simulink model "robot_echant_etu"  (R2022a)
settings: Solver=VariableStepAuto  StartTime=0.0  StopTime=10.0  RelTol=1e-3
values from neighbouring files (symbols this model uses):
  K = -place(A,B,[-136.4009, -2.6408, -3.5890, -5.9800])    [matrices.m]    (also in simu_robot_etu.m = [0.6700 19.9055 1.0747  1.9614])
  ue = 0    [simu_robot_etu.m]
  x0 = [0 pi/10 0 0]    [simu_robot_etu.m]
  xe = [0 0 0 0]'    [simu_robot_etu.m]
undefined symbols (not defined in the file or in its folder): DiscIntNeverNeededParam, X0
libraries: simulink x1
settings Model: Creator=melallem  LastModifiedBy=elgue
settings DebuggingCC: UnconnectedInputMsg=warning  UnconnectedOutputMsg=warning  UnconnectedLineMsg=warning
settings RTWCC: DLArmComputeVersion=19.05

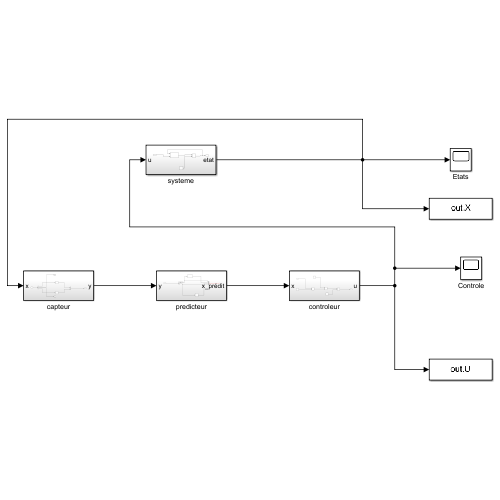
[thumbnail: Simulink's stored preview of the top-level diagram]
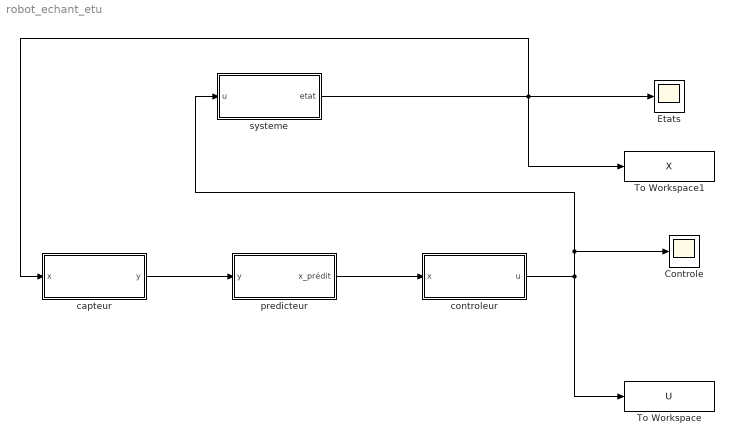
== system robot_echant_etu ==
  Controle : Scope
  Etats : Scope
  To Workspace : ToWorkspace  VariableName=U  SaveFormat=Timeseries  SampleTime=-1
  To Workspace1 : ToWorkspace  VariableName=X  SaveFormat=Timeseries  SampleTime=-1
  capteur : Subsystem
  controleur : Subsystem
  predicteur : Subsystem
  systeme : Subsystem
  wires:
  controleur/1(u) -> To Workspace/1, systeme/1(u), Controle/1
  predicteur/1(x_prédit) -> controleur/1(x)
  capteur/1(y) -> predicteur/1(y)
  systeme/1(etat) -> To Workspace1/1, capteur/1(x), Etats/1

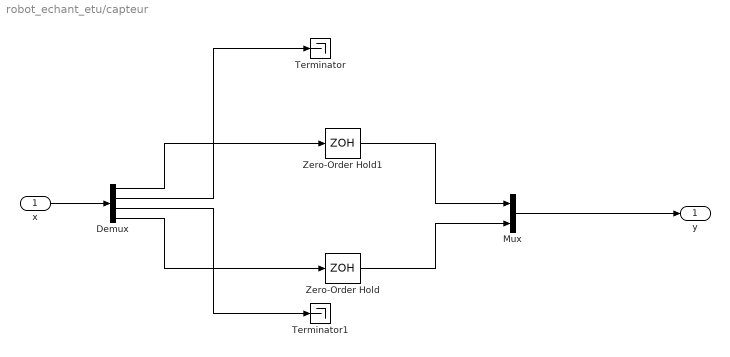
== system robot_echant_etu/capteur ==
  x : Inport
  Demux : Demux
  Mux : Mux  Inputs=2
  Terminator : Terminator
  Terminator1 : Terminator
  Zero-Order Hold : ZeroOrderHold  SampleTime=-1
  Zero-Order Hold1 : ZeroOrderHold  SampleTime=-1
  y : Outport
  wires:
  x/1 -> Demux/1
  Zero-Order Hold1/1 -> Mux/1
  Zero-Order Hold/1 -> Mux/2
  Mux/1 -> y/1
  Demux/2 -> Terminator/1
  Demux/3 -> Terminator1/1
  Demux/4 -> Zero-Order Hold/1
  Demux/1 -> Zero-Order Hold1/1

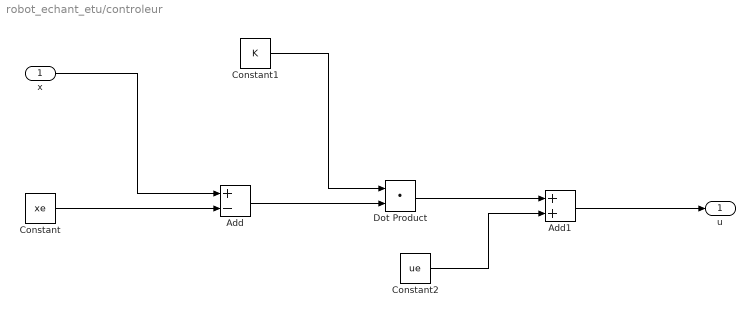
== system robot_echant_etu/controleur ==
  x : Inport
  Add : Sum  Inputs=+-
  Add1 : Sum
  Constant : Constant  Value=xe
  Constant1 : Constant  Value=K
  Constant2 : Constant  Value=ue
  Dot Product : DotProduct  OutDataTypeStr=Inherit: Inherit via internal rule
  u : Outport
  wires:
  x/1 -> Add/1
  Constant/1 -> Add/2
  Constant1/1 -> Dot Product/1
  Add/1 -> Dot Product/2
  Dot Product/1 -> Add1/1
  Constant2/1 -> Add1/2
  Add1/1 -> u/1

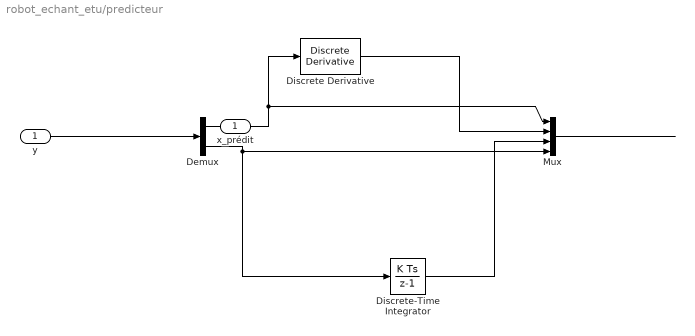
== system robot_echant_etu/predicteur ==
  y : Inport
  Demux : Demux  Outputs=2
  Discrete Derivative : simulink/Discrete/Discrete Derivative  gainval=1.0  ICPrevScaledInput=0.0  OutMin=[]  OutMax=[]  OutDataType=fixdt(1, 16)  OutScaling=2^-10  DoSatur=off
  Discrete-Time Integrator : DiscreteIntegrator  InitialCondition=X0(2)  SampleTime=-1  ICPrevOutput=DiscIntNeverNeededParam  ICPrevScaledInput=DiscIntNeverNeededParam
  Mux : Mux
  x_prédit : Outport
  wires:
  y/1 -> Demux/1
  Demux/1 -> Discrete Derivative/1, Mux/1
  Demux/2 -> Discrete-Time Integrator/1, Mux/4
  Discrete-Time Integrator/1 -> Mux/3
  Discrete Derivative/1 -> Mux/2
  Mux/1 -> ?

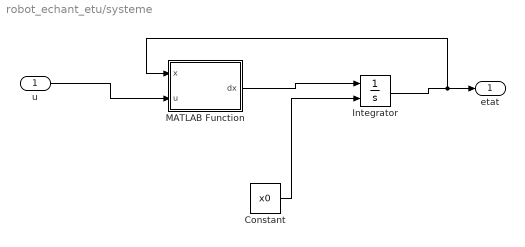
== system robot_echant_etu/systeme ==
  u : Inport
  Constant : Constant  Value=x0
  Integrator : Integrator  InitialConditionSource=external
  MATLAB Function : MATLAB Function  TreatAsAtomicUnit=on
  etat : Outport
  wires:
  u/1 -> MATLAB Function/2(u)
  MATLAB Function/1(dx) -> Integrator/1
  Constant/1 -> Integrator/2
  Integrator/1 -> MATLAB Function/1(x), etat/1

== matlab function robot_echant_etu/systeme/MATLAB Function ==
  data: x input; u input; dx output
function dx = fcn(x,u)
dx=fonction(x,u); 
end
